simulink model "oringin_revise_2_28_test_path_L_F"  (R2019a)
settings: Solver=VariableStepAuto  StartTime=0.0  StopTime=inf  RelTol=1e-3
values from neighbouring files (symbols this model uses):
  ki = 0    [revise_2_28_path_dd_L_F.m]
  lam = 1.25    [revise_2_28_path_dd_L_F.m]
undefined symbols (not defined in the file or in its folder): Angular, kp, Linear
libraries: robotlib x3, sharedtransform x1, simulink x1
settings Model: Creator=root  LastModifiedBy=root

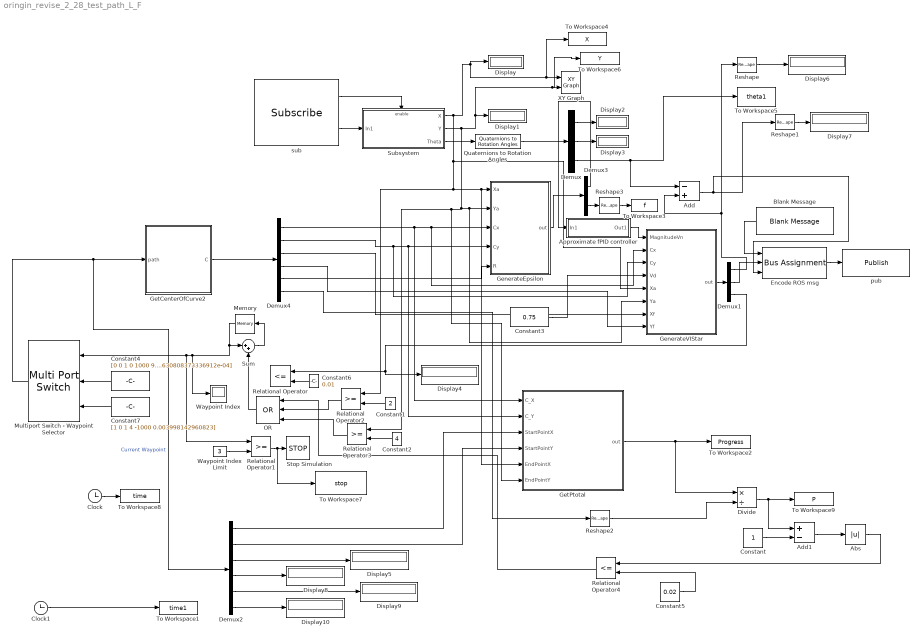
== system oringin_revise_2_28_test_path_L_F ==
  Abs : Abs
  Add : Sum  Inputs=-+
  Add1 : Sum  Inputs=+-
  Approximate fPID controller : Subsystem  mask{Kp=kp, II=[ki lam], DD=[0 0.5], N=5, ww=[1e-3 1e3], kFilter=Oustaloup filter}
      mask prompts: Kp "Proportional Kp"; II "Integral [Ki lam]"; DD "Differentiation [Kd mu]"; N "Filter order"; ww "Interested frequency range [wb wh]"; kFilter "Types of the filter"
      mask init:
      | if isa(Kp,'fotf'), a=Kp;
      |    lam=a.nd; mu=a.nn; mu=mu(1)-lam; b=a.num;
      |    Kd=b(1); Kp=b(2); Ki=b(3);
      | else
      |    II=[II 1]; DD=[DD 1]; Ki=II(1); lam=II(2); Kd=DD(1); mu=DD(2);
      | end
      | key=0; if mu>=1, key=1; end
      mask TypeOptions kFilter: Oustaloup filter | Modified Oustaloup filter
      mask Display: disp('Fractional-order\nPID controller')
  Blank Message : robotlib/Blank Message  messageClass=Message  entityType=geometry_msgs/Twist  messageType=geometry_msgs/Twist  SampleTime=inf
      settings: SourceProductBaseCode=RO
  Clock : Clock
  Clock1 : Clock
  Constant : Constant
  Constant1 : Constant  Value=2
  Constant2 : Constant  Value=4
  Constant3 : Constant  Value=0.75
  Constant4 : Constant  Value=[0 0 1 0 1000 9.630808373336912e-04]
  Constant5 : Constant  Value=0.02
  Constant6 : Constant  Value=0.01
  Constant7 : Constant  Value=[1 0 1 4 -1000 0.003998142960823]
  Demux : Demux  Outputs=3
  Demux1 : Demux  Outputs=3
  Demux2 : Demux  Outputs=6
  Demux3 : Demux  Outputs=2
  Demux4 : Demux  Outputs=6
  Display{,1..10} (11 alike) : Display
  Divide : Product  Inputs=*/
  Encode ROS msg : BusAssignment  AssignedSignals=Linear.X,Angular.Z
  GenerateEpsilon : MATLAB Function  TreatAsAtomicUnit=on
  GenerateVIStar : MATLAB Function  TreatAsAtomicUnit=on
  GetCenterOfCurve2 : MATLAB Function  TreatAsAtomicUnit=on
  GetPtotal : MATLAB Function  TreatAsAtomicUnit=on
  Memory : Memory  InitialCondition=1
  Multiport Switch - Waypoint Selector : MultiPortSwitch  Inputs=2  DiagnosticForDefault=Warning
  OR : Logic  Operator=OR  Inputs=3  IconShape=distinctive  AllPortsSameDT=off  OutDataTypeStr=boolean
  Quaternions to Rotation Angles : sharedtransform/Quaternions to Rotation Angles  rotationOrder=ZYX  aMode=aMode
      settings: SourceProductBaseCode=AE
  Relational Operator : RelationalOperator  Operator=<=  OutDataTypeStr=boolean  RndMeth=Simplest
  Relational Operator1 : RelationalOperator  OutDataTypeStr=boolean  RndMeth=Simplest
  Relational Operator2 : RelationalOperator  OutDataTypeStr=boolean  RndMeth=Simplest
  Relational Operator3 : RelationalOperator  OutDataTypeStr=boolean  RndMeth=Simplest
  Relational Operator4 : RelationalOperator  Operator=<=  OutDataTypeStr=boolean  RndMeth=Simplest
  Reshape{,1..3} (4 alike) : Reshape
  Stop Simulation : Stop
  Subsystem : Subsystem
  Sum : Sum  Inputs=|++
  To Workspace1 : ToWorkspace  VariableName=time1  SampleTime=0.05
  To Workspace2 : ToWorkspace  VariableName=Progress  SampleTime=0.05
  To Workspace3 : ToWorkspace  VariableName=f  SaveFormat=Timeseries  SampleTime=0.05
  To Workspace4 : ToWorkspace  VariableName=X  SampleTime=0.05
  To Workspace5 : ToWorkspace  VariableName=theta1  SaveFormat=Timeseries  SampleTime=-1
  To Workspace6 : ToWorkspace  VariableName=Y  SampleTime=0.05
  To Workspace7 : ToWorkspace  VariableName=stop  SaveFormat=Timeseries  SampleTime=-1
  To Workspace8 : ToWorkspace  VariableName=time  SampleTime=0.05
  To Workspace9 : ToWorkspace  VariableName=P  SampleTime=0.05
  Waypoint Index : Display
  Waypoint Index Limit : Constant  Value=3
  XY Graph : simulink/Sinks/XY Graph  xmin=-3  xmax=15  ymin=-3  ymax=10  st=-1
  pub : robotlib/Publish  topicSource=Select from ROS network  topic=/cmd_vel  messageType=geometry_msgs/Twist  messageQueueLength=100
      settings: SourceProductBaseCode=RO
  sub : robotlib/Subscribe  topicSource=Select from ROS network  topic=/odom  messageType=nav_msgs/Odometry  sampleTime=0.01  messageQueueLength=100
      settings: SourceProductBaseCode=RO
  wires:
  Divide/1 -> To Workspace9/1, Add1/1
  Reshape2/1 -> Divide/2
  Demux4/3 -> GenerateVIStar/7(Xf)
  Encode ROS msg/1 -> pub/1
  Demux2/2 -> GetPtotal/4(StartPointY)
  Reshape1/1 -> Display7/1
  Constant2/1 -> Relational Operator3/2
  Demux2/4 -> Display8/1
  Relational Operator4/1 -> OR/1
  Demux2/5 -> Display9/1
  Demux4/4 -> GenerateVIStar/8(Yf)
  Sum/1 -> Memory/1
  Relational Operator1/1 -> To Workspace7/1, Stop Simulation/1
  Demux4/5 -> GenerateEpsilon/5(R)
  sub/2 -> Subsystem/1(In1)
  Demux/1 -> Display2/1
  Constant5/1 -> Relational Operator4/2
  Relational Operator2/1 -> OR/2
  Demux1/2 -> Encode ROS msg/2
  Demux4/2 -> GenerateVIStar/3(Cy), GetPtotal/2(C_Y), GenerateEpsilon/4(Cy)
  Demux1/1 -> Reshape/1, Add/2
  Demux3/2 -> Reshape3/1
  Demux2/1 -> GetPtotal/3(StartPointX)
  Constant4/1 -> Multiport Switch - Waypoint Selector/2
  Reshape3/1 -> To Workspace3/1
  OR/1 -> Sum/2
  Demux1/3 -> Relational Operator/1, Display4/1
  Clock/1 -> To Workspace8/1
  Quaternions to Rotation Angles/1 -> Demux/1
  sub/1 -> Subsystem/Enable
  GetCenterOfCurve2/1(C) -> Demux4/1
  Demux2/3 -> Display5/1
  Constant1/1 -> Relational Operator2/2
  Subsystem/1(X) -> GetPtotal/5(EndPointX), GenerateEpsilon/1(Xa), Relational Operator2/1, GenerateVIStar/5(Xa), To Workspace4/1, XY Graph/1, Display/1
  Blank Message/1 -> Encode ROS msg/1
  Add/1 -> Encode ROS msg/3, Reshape1/1
  GenerateVIStar/1(out) -> Demux1/1
  Demux4/6 -> Reshape2/1
  Add1/1 -> Abs/1
  Approximate fPID controller/1(Out1) -> GenerateVIStar/1(MagnitudeVn)
  Constant/1 -> Add1/2
  Reshape/1 -> Display6/1
  Constant6/1 -> Relational Operator/2
  GetPtotal/1(out) -> Divide/1, To Workspace2/1
  Subsystem/3(Theta) -> Quaternions to Rotation Angles/1
  Demux3/1 -> Approximate fPID controller/1(In1)
  GenerateEpsilon/1(out) -> Demux3/1
  Demux/3 -> Add/1, To Workspace5/1
  Waypoint Index Limit/1 -> Relational Operator1/2
  Demux2/6 -> Display10/1
  Clock1/1 -> To Workspace1/1
  Demux/2 -> Display3/1
  Subsystem/2(Y) -> Relational Operator3/1, GetPtotal/6(EndPointY), GenerateVIStar/6(Ya), GenerateEpsilon/2(Ya), Display1/1, To Workspace6/1, XY Graph/2
  Multiport Switch - Waypoint Selector/1 -> Demux2/1, GetCenterOfCurve2/1(path)  "Current Waypoint"
  Constant7/1 -> Multiport Switch - Waypoint Selector/3
  Constant3/1 -> GenerateVIStar/4(Vd)
  Relational Operator3/1 -> OR/3
  Memory/1 -> Multiport Switch - Waypoint Selector/1, Relational Operator1/1, Waypoint Index/1, Sum/1
  Abs/1 -> Relational Operator4/1
  Demux4/1 -> GetPtotal/1(C_X), GenerateVIStar/2(Cx), GenerateEpsilon/3(Cx)

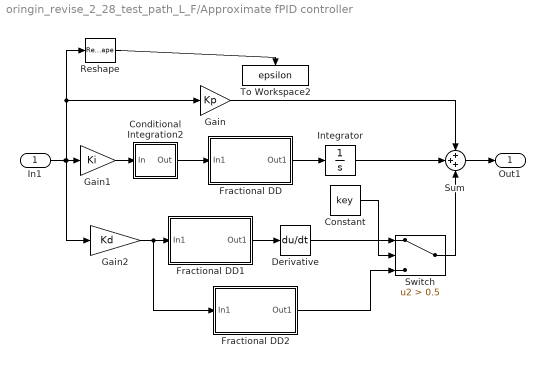
== system oringin_revise_2_28_test_path_L_F/Approximate fPID controller ==
  In1 : Inport
  Conditional Integration2 : Subsystem
  Constant : Constant  Value=key
  Derivative : Derivative
  Fractional DD : Subsystem  mask{gam=1-lam, ww=ww, n=N}
      mask prompts: gam "Derivative order gamma"; ww "Frequency range [wb,wh]"; n "Apprixmation order"
      mask init:
      | wb=ww(1); wh=ww(2); G=ousta_fod(gam,n,wb,wh); 
      | num=G.num{1}; den=G.den{1}; T=1/wh; str='Fractional\n';
      | if isnumeric(gam)
      | 	if gam>0, str=[str, 'Der  s^' num2str(gam) ];
      | 	else, str=[str, 'Int  s^{' num2str(gam) '}']; end
      | else, str=[str, 'Der  s^gam']; end
      mask Display: disp(str)
  Fractional DD1 : Subsystem  mask{gam=mu-1, ww=ww, n=N}
      mask prompts: gam "Derivative order gamma"; ww "Frequency range [wb,wh]"; n "Apprixmation order"
      mask init: same as oringin_revise_2_28_test_path_L_F/Approximate fPID controller/Fractional DD
      mask Display: disp(str)
  Fractional DD2 : Subsystem  mask{gam=mu, ww=ww, n=N}
      mask prompts: gam "Derivative order gamma"; ww "Frequency range [wb,wh]"; n "Apprixmation order"
      mask init: same as oringin_revise_2_28_test_path_L_F/Approximate fPID controller/Fractional DD
      mask Display: disp(str)
  Gain : Gain  Gain=Kp
  Gain1 : Gain  Gain=Ki
  Gain2 : Gain  Gain=Kd
  Integrator : Integrator
  Reshape : Reshape
  Sum : Sum  Inputs=+++
  Switch : Switch  Criteria=u2 > Threshold  Threshold=0.5
  To Workspace2 : ToWorkspace  VariableName=epsilon  SampleTime=0.05
  Out1 : Outport
  wires:
  Constant/1 -> Switch/2
  Switch/1 -> Sum/3
  Fractional DD2/1(Out1) -> Switch/3
  Derivative/1 -> Switch/1
  Gain2/1 -> Fractional DD1/1(In1), Fractional DD2/1(In1)
  Gain/1 -> Sum/1
  Fractional DD1/1(Out1) -> Derivative/1
  Sum/1 -> Out1/1
  Integrator/1 -> Sum/2
  Fractional DD/1(Out1) -> Integrator/1
  Reshape/1 -> To Workspace2/1
  In1/1 -> Gain1/1, Gain2/1, Gain/1, Reshape/1
  Gain1/1 -> Conditional Integration2/1(In)
  Conditional Integration2/1(Out) -> Fractional DD/1(In1)

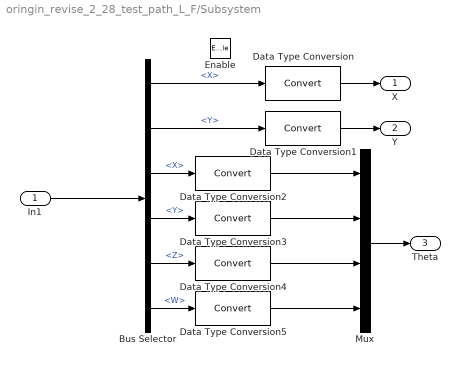
== system oringin_revise_2_28_test_path_L_F/Subsystem ==
  In1 : Inport
  Enable : EnablePort
  Bus Selector : BusSelector  OutputSignals=Pose.Pose.Position.X,Pose.Pose.Position.Y,Pose.Pose.Orientation.X,Pose.Pose.Orientation.Y,Pose.Pose.Orientation.Z,Pose.Pose.Orientation.W
  Data Type Conversion{,1..5} (6 alike) : DataTypeConversion
  Mux : Mux
  X : Outport
  Y : Outport  Port=2
  Theta : Outport  Port=3
  wires:
  Bus Selector/1 -> Data Type Conversion/1  "<X>"
  In1/1 -> Bus Selector/1
  Data Type Conversion/1 -> X/1
  Bus Selector/2 -> Data Type Conversion1/1  "<Y>"
  Data Type Conversion1/1 -> Y/1
  Data Type Conversion2/1 -> Mux/1
  Bus Selector/3 -> Data Type Conversion2/1  "<X>"
  Bus Selector/4 -> Data Type Conversion3/1  "<Y>"
  Bus Selector/5 -> Data Type Conversion4/1  "<Z>"
  Bus Selector/6 -> Data Type Conversion5/1  "<W>"
  Data Type Conversion5/1 -> Mux/4
  Data Type Conversion4/1 -> Mux/3
  Data Type Conversion3/1 -> Mux/2
  Mux/1 -> Theta/1

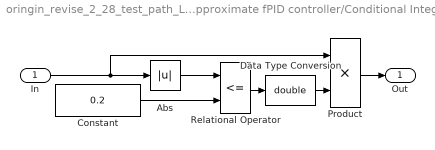
== system oringin_revise_2_28_test_path_L_F/Approximate fPID controller/Conditional Integration2 ==
  In : Inport
  Abs : Abs  SaturateOnIntegerOverflow=on
  Constant : Constant  Value=0.2
  Data Type Conversion : DataTypeConversion  OutDataTypeStr=double
  Product : Product  SaturateOnIntegerOverflow=on  RndMeth=Zero  InputSameDT=on  OutDataTypeStr=Inherit: Same as first input
  Relational Operator : RelationalOperator  Operator=<=  RndMeth=Nearest  InputSameDT=on
  Out : Outport
  wires:
  Data Type Conversion/1 -> Product/2
  Relational Operator/1 -> Data Type Conversion/1
  Abs/1 -> Relational Operator/1
  Constant/1 -> Relational Operator/2
  Product/1 -> Out/1
  In/1 -> Abs/1, Product/1

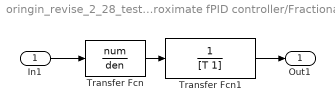
== system oringin_revise_2_28_test_path_L_F/Approximate fPID controller/Fractional DD ==
  In1 : Inport
  Transfer Fcn : TransferFcn  Numerator=num  Denominator=den
  Transfer Fcn1 : TransferFcn  Numerator=1  Denominator=[T 1]
  Out1 : Outport
  wires:
  Transfer Fcn1/1 -> Out1/1
  Transfer Fcn/1 -> Transfer Fcn1/1
  In1/1 -> Transfer Fcn/1

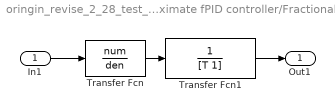
== system oringin_revise_2_28_test_path_L_F/Approximate fPID controller/Fractional DD1 ==
  In1 : Inport
  Transfer Fcn : TransferFcn  Numerator=num  Denominator=den
  Transfer Fcn1 : TransferFcn  Numerator=1  Denominator=[T 1]
  Out1 : Outport
  wires:
  In1/1 -> Transfer Fcn/1
  Transfer Fcn/1 -> Transfer Fcn1/1
  Transfer Fcn1/1 -> Out1/1

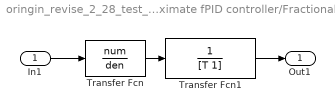
== system oringin_revise_2_28_test_path_L_F/Approximate fPID controller/Fractional DD2 ==
  In1 : Inport
  Transfer Fcn : TransferFcn  Numerator=num  Denominator=den
  Transfer Fcn1 : TransferFcn  Numerator=1  Denominator=[T 1]
  Out1 : Outport
  wires:
  Transfer Fcn1/1 -> Out1/1
  Transfer Fcn/1 -> Transfer Fcn1/1
  In1/1 -> Transfer Fcn/1

== matlab function oringin_revise_2_28_test_path_L_F/GetPtotal ==
  data: out output; C_X input; C_Y input; StartPointX input; StartPointY input; EndPointX input; EndPointY input
function out = GetPtotal(C_X, C_Y,StartPointX,StartPointY, EndPointX, EndPointY)

% Based on the Center, StartPoint and EndPoint this function computes the 
% Total Progress along the path in degrees.

% Programmer : Vikas Bahl
% Written on : 5th February 2001


% This is the distance from the center to the start point.
dCrToSp     = sqrt( (C_X - StartPointX)^2 + (C_Y - StartPointY)^2 );
% This is the distance from the center to the end point. 
dCrToEp     = sqrt( (C_X - EndPointX)^2 + (C_Y - EndPointY)^2 );
% This is the distance from the start point to the end point.
dSpToEp     = sqrt( (StartPointX - EndPointX)^2 + (StartPointY - EndPointY)^2 );

MyQuantity  = (dCrToSp^2 + dCrToEp^2 - dSpToEp^2) / (2*dCrToSp*dCrToEp);
if ( MyQuantity > 1.0 )
MyQuantity = 1.0;
else
MyQuantity = MyQuantity;
end
% Define the Total Progress Angle as 'PTotal' and compute it:
PTotal      = acos( MyQuantity );

out         = PTotal;

== matlab function oringin_revise_2_28_test_path_L_F/GenerateVIStar ==
  data: MagnitudeVn input; Cx input; Cy input; Vd input; Xa input; Ya input; out output; Xf input; Yf input
function out = GenerateVIStar( MagnitudeVn, ...
                               Cx,  Cy,  Vd, ... 
                               Xa,  Ya,  Xf, Yf)

% The function PathTrack is called by the Sensor Motion Scheduler (SMS).
% Parameters :
%
% Cx         : X Coordinate of the center.              Unit m
% Cy         : Y Coordinate of the center.              Unit m
% R          : Radius of the arc Path.                  Unit m
% Vd         : Desired Velocity.                        Unit m/sec
% Xa         : Actual X Position (from Feedback).       Unit m
% Ya         : Actual Y Position (from Feedback).       Unit m
%
% Output's   : 
%
% ViStar     : Desired Inertial Velocity (2x1 Vector).  Unit m/sec

% Programmer : Vikas Bahl
% Written on : 5th February 2001
if Cy > 10
%     rVector   = [0; -Ya];
%     Norm_r    = norm( rVector, 2 );
%     
% % Compute the Normal Velocity (Vn) in m/sec.
%     Vn        = MagnitudeVn * ( rVector / Norm_r );
    
% We follow the following steps to get the Tangential Velocity (Vt) in m/sec.
  quantity      = Vd - abs( MagnitudeVn );
  if ( quantity < 0 )
    quantity  = 0;
  
  else
    quantity  = quantity;

  end
% Vt            = (quantity / Norm_r) * [ abs(Ya); 0];
omga          =  atan(MagnitudeVn/quantity);

else
     rVector   = [1-Xa; 0];
    Norm_r    = norm( rVector, 2 );
    
    
% Compute the Normal Velocity (Vn) in m/sec.
    Vn        = abs(MagnitudeVn) * ( rVector / Norm_r );
    quantity      = Vd - abs( MagnitudeVn );
  if ( quantity < 0 )
    quantity  = 0;
  
  else
    quantity  = quantity;

  end
  Vt            = (quantity / Norm_r) * [0; abs(Xa-1)];

PreViStar     = Vt + Vn;
NormPreViStar = sqrt(PreViStar(1)^2 + PreViStar(2)^2);
X_X=[abs(PreViStar(1)), 0];
acos_value = (dot(PreViStar, X_X)/NormPreViStar);
if acos_value > 1
    acos_value = 1;
elseif acos_value < -1
    acos_value = -1;
else
    acos_value = acos_value;
end

  if PreViStar(2) >= 0
    omga          =  acos(acos_value);
  else 
    omga          =  -acos(acos_value);
  end
end
%omga      =  atan(MagnitudeVn/quantity);


dist = sqrt((Xf-Xa)^2+(Yf-Ya)^2);

out = [omga Vd dist];

== matlab function oringin_revise_2_28_test_path_L_F/GenerateEpsilon ==
  data: Xa input; Ya input; out output; Cx input; Cy input; R input
function out = GenerateEpsilon( Xa, Ya, Cx, Cy, R)
%
%                                                                                   
% Function used by the control system: 
%          It Generates Epsilon.
%
% Parameters Used:
%           Cx      = X coordinate of the center of the curve. Unit m
%           Cy      = Y coordinate of the center of the curve. Unit m
%           R       = Radius of the curve.(Infinite in case of Translate).
%           X       = The actual X position (from the simulink model). Unit m
%           Y       = The actual Y position (from the simulink model). Unit m
% Based on the above parameters this function computes Epsilon:
%           Epsilon = abs(R) - Norm_r
%           where Norm_r is the 2-Norm of the rVector = [ X-Cx 
%                                                         Y-Cy ] 
%

% Programmer : Vikas Bahl.
% Written on : 19th February 2001.

rVector       = [ Xa - Cx ; Ya - Cy ];
Norm_r        = norm( rVector, 2 );

%epsilon      = ( abs(R) - Norm_r );
if Cx         < 1
    epsilon   = Ya;
else
    epsilon   = Xa - 1;
end

f             = abs(R^2 - (R-epsilon)^2); 
out           = [epsilon f];

== matlab function oringin_revise_2_28_test_path_L_F/GetCenterOfCurve2 ==
  data: C output; path input
function C = GetCenterOfCurve( path )

% This function takes the start point , the end point and the radius provided by the user
% and computes the center of the curve.
% The start point and the end points are 2x1 Vectors represented as: [X_S;Y_s] and [X_f;Y_f]
% respectively.

% Programmer:	Vikas Bahl
% Written On:	11th February 2001.

x_s    = path(1); 
y_s    = path(2);
x_f    = path(3); 
y_f    = path(4);
radius = path(5);
ptotal = path(6);


%If the Start point is the same as the End point then we have an error.
if ( (x_s == x_f) && (y_s == y_f) )
   error('Data not valid: start point should be different with the final point.');
end

% If the specified radius is less than half the distance between the line joining the starting
% and the ending point then we have an error again.
x_difference  = x_f-x_s;
y_difference  = y_f-y_s;
line_distance = sqrt(x_difference^2 + y_difference^2);
if (abs(radius) < 0.5*line_distance)
   error('The given Radius not valid: radius is too small');
end

% Now we find the center point of the line joining the start point and the end point
line_center_x = (x_f + x_s)/2;
line_center_y = (y_f + y_s)/2;

% Once the center point of the line joining the start point and the end point is found
% we want to calculate the vertical distance from that point to the center of the arc.
vertDistToCenter = GetTriangleSideLength(abs(radius), 0.5 * line_distance);

% First we treat the special cases,i.e., if the line joining the start point and the end point
% is at 0 degrees,i.e., either X_s = X_f or Y_s = Y_f.
if (x_s == x_f)
   c_y = line_center_y; % the center point of start and end    	
   
   % determine the x_offset   	
   if ((y_f - y_s) * radius > 0) 		
      % the center is at the left of the center point of the line   		
      c_x = x_s - vertDistToCenter; 
      
   else 		
      % the center is at the right of the center point of the line
      c_x = x_s + vertDistToCenter;
   end
   
   C = [c_x c_y x_f y_f abs(radius) ptotal];
   
   return
   
elseif(y_s == y_f)
   c_x = line_center_x; % the center point of start and end
   
   % determine the y_offset
   if ((x_f - x_s)*radius > 0)
      % the center is above the center point of the line
      c_y = y_s + vertDistToCenter;
      
   else
      % the center is below the center point of the line
      c_y = y_s - vertDistToCenter;
   end
   
   C = [c_x c_y x_f y_f abs(radius) ptotal];
   
   return
end
% The general Case  
tanOfLine  = (y_f - y_s)/(x_f - x_s); 
tanOfRLine = -1/tanOfLine;  

% cos value    
distance   = vertDistToCenter/(sqrt(1 + tanOfRLine * tanOfRLine)); 
c_x1       = line_center_x + distance; 
c_x2       = line_center_x - distance;  

% from the line function get y value    
a          = tanOfRLine;  
b          = line_center_y - a * line_center_x; 
c_y1       = a * c_x1 + b; 
c_y2       = a * c_x2 + b;          

% determine which one is the true circle center assume the circle center is at c_x1 and c_y1   
% using p1 * p2 to determine whether it is Ok    

judgeXY    = (x_s - c_x1) * (y_f - c_y1) - (x_f - c_x1) * (y_s - c_y1);  

if (judgeXY * radius > 0) 	
   c_x     = c_x1; 	
   c_y     = c_y1; 
else  	
   c_x     = c_x2; 	
   c_y     = c_y2; 
end
C = [c_x c_y x_f y_f abs(radius) ptotal];
